simulink model "Operation_math"  (R2021a)
settings: Solver=VariableStepAuto  StartTime=0.0  StopTime=10.0  RelTol=1e-3
settings Model: Creator=Aula  LastModifiedBy=Aula

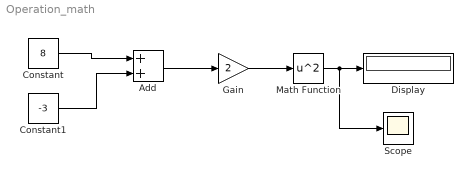
== system Operation_math ==
  Add : Sum
  Constant : Constant  Value=8
  Constant1 : Constant  Value=-3
  Display : Display
  Gain : Gain  Gain=2
  Math Function : Math  Operator=square  SaturateOnIntegerOverflow=on
  Scope : Scope
  wires:
  Constant/1 -> Add/1
  Constant1/1 -> Add/2
  Add/1 -> Gain/1
  Gain/1 -> Math Function/1
  Math Function/1 -> Scope/1, Display/1
